simulink model "Tutorial_1_3"  (R2023a)
settings: Solver=FixedStepAuto  StartTime=0.0  StopTime=10.0  FixedStep=1e-3  RelTol=1e-3  EnableMultiTasking=on
libraries: frdmk64flib x4
settings Model: ExtModeTrigDuration=5  Creator=sadeg  LastModifiedBy=sadeg
settings OptimizationCC: EnhancedBackFolding=on  PassReuseOutputArgsAs=Individual arguments  ZeroExternalMemoryAtStartup=off  ZeroInternalMemoryAtStartup=off  MaxStackSize=64  OptimizeBlockOrder=speed  DifferentSizesBufferReuse=on  OptimizationCustomize=off  EfficientTunableParamExpr=on
settings DebuggingCC: ParameterTunabilityLossMsg=error
settings HardwareCC: ProdBitPerPointer=32  ProdBitPerSizeT=32  ProdBitPerPtrDiffT=32  ProdLargestAtomicInteger=Long  ProdLargestAtomicFloat=Double  ProdWordSize=32  ProdHWDeviceType=ARM Compatible->ARM Cortex  UseEmbeddedCoderFeatures=off
settings SFSimCC: MATLABDynamicMemAlloc=off
settings RTWCC: Description=Embedded Coder  SystemTargetFile=ert.tlc  HardwareBoard=NXP FRDM-K64F  TLCOptions="-aInlineSetEventsForThisBaseRateFcn=TLC_FALSE -aSuppressMultiTaskScheduler=TLC_FALSE  -aRateBasedStepFcn=0"  TemplateMakefile=ert_default_tmf  Toolchain=GNU Tools for ARM Embedded Processors
settings CodeAppCC: ForceParamTrailComments=on  IgnoreCustomStorageClasses=off  OperatorAnnotations=on  SimulinkDataObjDesc=on  SFDataObjDesc=on  InsertBlockDesc=on
settings ERTTargetCC: SupportNonInlinedSFcns=on  ExtModeTransport=4  ExtModeMexFile=sendToCommService

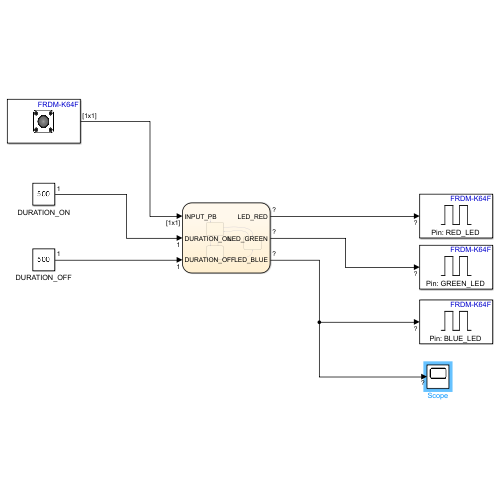
[thumbnail: Simulink's stored preview of the top-level diagram]
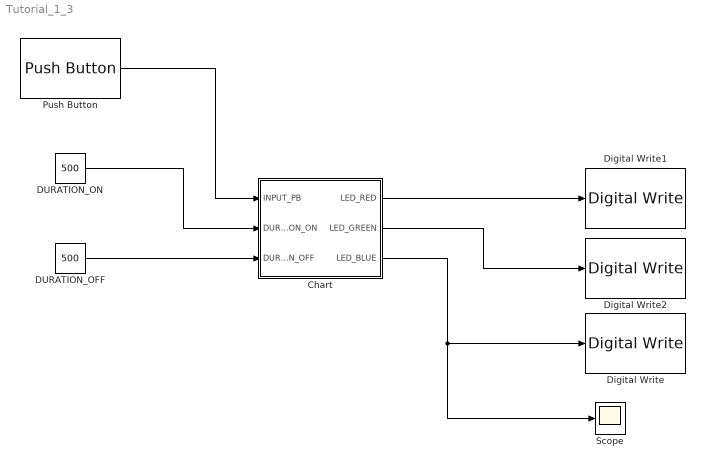
== system Tutorial_1_3 ==
  Chart : Stateflow chart  TreatAsAtomicUnit=on
      settings: PortSchema="{\"entries\":[{\"content\":{\"sides\":[{\"content\":{\"connectorIds\":[\"In1\",\"In2\",\"In3\"]},\"type\":\"ConnectorPlacement.EquallySpacedRectSide\",\"uuid\":\"03af61af-7cb8-4be0-af6f-2114e055ec24\"},{\"content\":{\"connectorIds\":[\"Out3\",\"Out1\",\"Out2\"],\"side\":\"RIGHT\"},\"type\":\"ConnectorPlacement.EquallySpacedRectSide\",\"uuid\":\"f00e0b89-c4eb-4fa3-a72e-3df85b5d4963\"},{\"content\":{\"side\":\"TOP\"},\"type\":\"ConnectorPlacement.EquallySpacedRectSide\",\"uuid\":\"62265664-fc2c-4b7b-8595-4678a4c4b375\"}]},\"type\":\"ConnectorPlacement.EquallySpacedConnector\",\"uuid\":\"a4b8bb8d-837d-45a6-af13-e6335961bb51\"}],\"packageUris\":[\"http://schema.mathworks.com/mf0/Connector/R2020b\"],\"version\":\"1.0\"}"
  DURATION_OFF : Constant  Value=500  OutDataTypeStr=int16
  DURATION_ON : Constant  Value=500  OutDataTypeStr=int16
  Digital Write : frdmk64flib/Digital Write  Whichpin=BLUE_LED
  Digital Write1 : frdmk64flib/Digital Write  Whichpin=RED_LED
  Digital Write2 : frdmk64flib/Digital Write  Whichpin=GREEN_LED
  Push Button : frdmk64flib/Push Button  Whichswitch=SW2  SampleTime1=-1
  Scope : Scope
  wires:
  DURATION_ON/1 -> Chart/2(DURATION_ON)
  DURATION_OFF/1 -> Chart/3(DURATION_OFF)
  Push Button/1 -> Chart/1(INPUT_PB)
  Chart/3(LED_RED) -> Digital Write1/1
  Chart/1(LED_GREEN) -> Digital Write2/1
  Chart/2(LED_BLUE) -> Scope/1, Digital Write/1

== stateflow chart Tutorial_1_3/Chart ==
  state LED_ON
    entry:
    LED_STATE = true;
  state LED_OFF_FORCED
    entry:
    LED_STATE = false;
  state LED_OFF
    entry:
    LED_STATE = false;
  (default) -> LED_ON
  LED_ON -> LED_OFF_FORCED [order 2] : [INPUT_PB == 1]
  LED_OFF_FORCED -> LED_ON : [INPUT_PB == 0]
  LED_ON -> LED_OFF [order 1] : after(DURATION_ON, msec)
  LED_OFF -> LED_ON [order 1] : after(DURATION_OFF, msec)
  LED_OFF -> LED_OFF_FORCED [order 2] : [INPUT_PB == 1]
  data: LED_GREEN output; LED_BLUE output; INPUT_PB input; DURATION_ON input int16; DURATION_OFF input int16; LED_RED output boolean
